simulink model "roll_loop"  (R2020a)
settings: Solver=VariableStepAuto  StartTime=0.0  StopTime=1000  RelTol=1e-3
undefined symbols (not defined in the file or in its folder): AP, trans_func
libraries: aerolibactuator x1, slctrlblks x1
settings Model: Creator=nikhil  LastModifiedBy=VTOL_HYD
settings SFSimCC: CustomCodeUndefinedFunction=UseInterfaceOnly

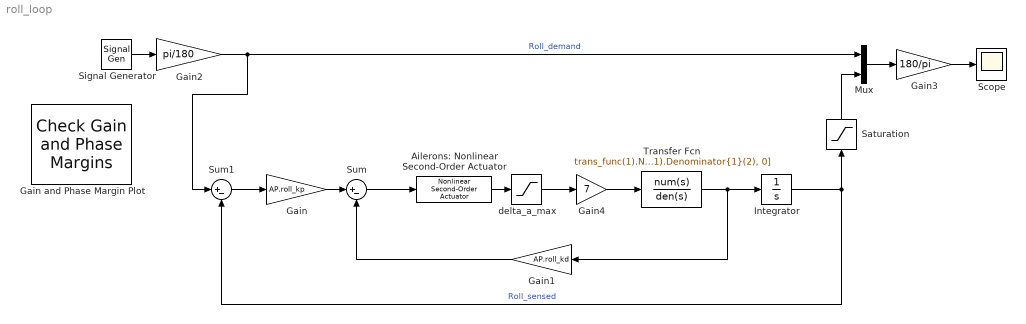
== system roll_loop ==
  Ailerons: Nonlinear Second-Order Actuator : aerolibactuator/Nonlinear Second-Order Actuator  wn_fin=200  z_fin=0.5  fin_max=20*pi/180  fin_min=-20*pi/180  fin_maxrate=500*pi/180  fin_act_0=0  fin_act_vel=0
      settings: SourceProductBaseCode=AE
  Gain : Gain  Gain=AP.roll_kp
  Gain and Phase Margin Plot : slctrlblks/Model Verification/Check Gain and Phase Margins  InstantiateOnLoad=on  SaveOperatingPoints=off  LinearizationIOs={'/Sum1', 1, 'in', 'on', '';'/Integrator', 1, 'out', 'on', ''}  LinearizeAt=SnapshotTimes  SnapshotTimes=[0,10,50,100,200,300,400,500,600,700,800,900,1000]  TriggerType=rising  SampleTime=auto  RateConversionMethod=zoh  PreWarpFreq=10  UseExactDelayModel=off  UseFullBlockNameLabels=off  UseBusSignalLabels=off  enabled=on  stopWhenAssertionFail=off  export=off  ViewDlgPos=[1 41 1920 963]  LaunchViewOnOpen=off  OpenViewOnLoad=off  FrequencyUnits=rad/s  MagnitudeUnits=dB  PhaseUnits=deg  TimeUnits=seconds  EnableMargins=off  GainMargin=[]  PhaseMargin=[]  PlotType=table  FeedbackSign=-1
      settings: SourceProductBaseCode=SD  SaveToWorkspace=off  SaveName=sys
  Gain1 : Gain  Gain=AP.roll_kd
  Gain2 : Gain  Gain=pi/180
  Gain3 : Gain  Gain=180/pi
  Gain4 : Gain  Gain=7
  Integrator : Integrator
  Mux : Mux  Inputs=2
  Saturation : Saturate  UpperLimit=7  LowerLimit=-7
  Scope : Scope
  Signal Generator : SignalGenerator  WaveForm=square  Amplitude=20  Frequency=.1  Units=rad/sec
  Sum : Sum  Inputs=|+-
  Sum1 : Sum  Inputs=|+-
  Transfer Fcn : TransferFcn  Numerator=trans_func(1).Numerator{1}  Denominator=[trans_func(1).Denominator{1}(1), trans_func(1).Denominator{1}(2), 0]
  delta_a_max : Saturate  UpperLimit=0.785  LowerLimit=-.785
  wires:
  Transfer Fcn/1 -> Gain1/1, Integrator/1
  Integrator/1 -> Sum1/2, Saturation/1  "Roll_sensed"
  Gain1/1 -> Sum/2
  Gain2/1 -> Sum1/1, Mux/1  "Roll_demand"
  Sum1/1 -> Gain/1
  Gain/1 -> Sum/1
  Saturation/1 -> Mux/2
  Signal Generator/1 -> Gain2/1
  Mux/1 -> Gain3/1
  Gain3/1 -> Scope/1
  Ailerons: Nonlinear Second-Order Actuator/1 -> delta_a_max/1
  Sum/1 -> Ailerons: Nonlinear Second-Order Actuator/1
  delta_a_max/1 -> Gain4/1
  Gain4/1 -> Transfer Fcn/1
